simulink model "Test_Model_HR12_2016"  (R2016b)
settings: Solver=FixedStepAuto  StartTime=0.0  StopTime=length(ipoint)  FixedStep=dt  RelTol=1e-3
values from neighbouring files (symbols this model uses):
  Cbx_cyl_fill_efy_intk_mfld_prs_atm_prs_cor_cho = true    [Calib_mdl_RSA.m]
  Cbx_cyl_fill_efy_opt_cho = false    [Calib_mdl_RSA.m]
  Cbx_cyl_fill_igr_opt_cho = false    [Calib_mdl_RSA.m]
  Cbx_ex_vvt_conf = true    [Calib_mdl_RSA.m]
  Cnx_cyl_fill_ex_mfld_prs_cor_cho = 0    [Cal_basic.m]
  Cnx_cyl_nr_conf = 3    [Cal_basic.m]
  Cxx_cyl_fill_efy_drv_max = 20    [Calib_mdl_RSA.m]
  Cxx_cyl_fill_efy_dyn_max = 0.15    [Calib_mdl_RSA.m]
  Cxx_cyl_fill_efy_dyn_min = 0    [Calib_mdl_RSA.m]
  Cxx_cyl_fill_efy_dz = 0.45    [Calib_mdl_RSA.m]
  Cxx_cyl_fill_efy_ovlp_angl = 66    [Calib_mdl_RSA.m]
  Cxx_cyl_fill_efy_vvt_ofs = 0    [Calib_mdl_RSA.m]
  Cxx_cyl_fill_trap_area_h_thd = 0.2    [Cal_basic.m]
  Cxx_cyl_fill_trap_area_l_thd = 0.1    [Cal_basic.m]
  Cxx_cyl_fill_trap_efy_dz_l_thd = 1    [Cal_basic.m]
  Cxx_cyl_fill_trap_efy_dz_neg_slop = -0.5    [Cal_basic.m]
  Cxx_cyl_fill_trap_efy_dz_pos_slop = 0.5    [Cal_basic.m]
  Cxx_cyl_fill_trap_vvt_ovlp_angl = 120    [Calib_mdl_RSA.m]
  Cxx_cyl_vol = 3.9961e-04*3    (= 0.00119883)    [Cal_basic.m]    (also in Calib_mdl_RSA.m = 0.00119900004938)
  Cxx_min_cyl_fill_mdl_ex_mfld_prs_rat_cor = 0    [Cal_basic.m]
  Nnx_eng_run_stt = 2    [Calib_mdl_RSA.m]
  Nxx_atm_kpa = 101.3    [Cal_basic.m]
  Nxx_k_degc = 273.15    [Cal_basic.m]
  Nxx_kilo_bas = 1000    [Cal_basic.m]
  Nxx_wht_pgc_j_kg = 287    [Cal_basic.m]
undefined symbols (not defined in the file or in its folder): Cxx_egr_spc_heat, Cxx_thr_spc_heat, docblock, MapFilling_Aspirated
libraries: AEMS_Standard_Library x78, simulink x2
(part 2 of 5)

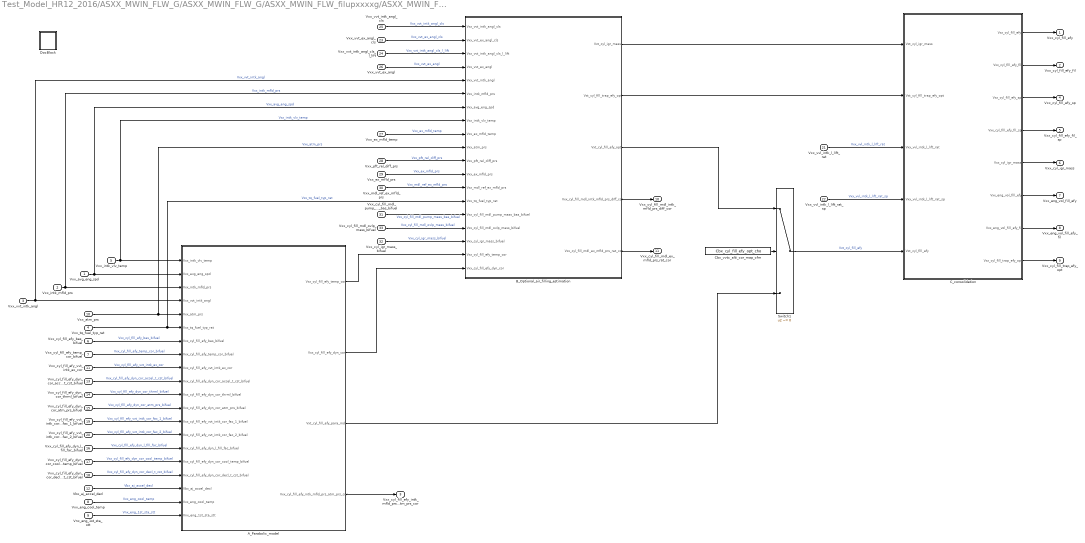
== system Test_Model_HR12_2016/ASXX_MWIN_FLW_G/ASXX_MWIN_FLW_G/ASXX_MWIN_FLW_filupxxxxg/ASXX_MWIN_FLW_filupxxxxg_10ms ==
  Vxx_avg_eng_spd : Inport  Interpolate=off
  Vxx_intk_mfld_prs : Inport  Port=2  Interpolate=off
  Vxx_vvt_intk_angl : Inport  Port=3  Interpolate=off
  Vxx_tq_fuel_typ_rat : Inport  Port=4  Interpolate=off
  Vxx_intk_vlv_temp : Inport  Port=5  Interpolate=off
  Vxx_cyl_fill_efy_bas_bifuel : Inport  Port=6  Interpolate=off
  Vxx_cyl_fill_efy_temp_cor_bifuel : Inport  Port=7  Interpolate=off
  Vxx_eng_cool_temp : Inport  Port=8  Interpolate=off
  Vnx_eng_1st_sta_stt : Inport  Port=9  Interpolate=off
  Vxx_atm_prs : Inport  Port=10  Interpolate=off
  Vxx_cyl_fill_efy_vvt_intk_ex_cor : Inport  Port=11  Interpolate=off
  Vbx_aj_accel_decl : Inport  Port=12  Interpolate=off
  Vxx_cyl_fill_efy_dyn_cor_accel_t_cst_bifuel : Inport  Port=13  Interpolate=off
  Vxx_cyl_fill_efy_dyn_cor_thrml_bifuel : Inport  Port=14  Interpolate=off
  Vxx_cyl_fill_efy_dyn_cor_atm_prs_bifuel : Inport  Port=15  Interpolate=off
  Vxx_cyl_fill_efy_dyn_l_fill_fac_bifuel : Inport  Port=16  Interpolate=off
  Vxx_cyl_fill_efy_dyn_cor_cool_temp_bifuel : Inport  Port=17  Interpolate=off
  Vxx_cyl_fill_efy_dyn_cor_decl_t_cst_bifuel : Inport  Port=18  Interpolate=off
  Vxx_cyl_fill_efy_vvt_intk_cor_fac_1_bifuel : Inport  Port=19  Interpolate=off
  Vxx_cyl_fill_efy_vvt_intk_cor_fac_2_bifuel : Inport  Port=20  Interpolate=off
  Vxx_vvl_intk_l_lift_rat : Inport  Port=21  Interpolate=off
  Vxx_vvl_intk_l_lift_rat_sp : Inport  Port=22  Interpolate=off
  Vxx_vvt_ex_angl_cls : Inport  Port=23  Interpolate=off
  Vxx_vvt_intk_angl_cls_l_lift : Inport  Port=24  Interpolate=off
  Vxx_vvt_intk_angl_cls : Inport  Port=25  Interpolate=off
  Vxx_vvt_ex_angl : Inport  Port=26  Interpolate=off
  Vxx_ex_mfld_temp : Inport  Port=27  Interpolate=off
  Vxx_pft_rel_diff_prs : Inport  Port=28  Interpolate=off
  Vxx_ex_mfld_prs : Inport  Port=29  Interpolate=off
  Vxx_mdl_ref_ex_mfld_prs : Inport  Port=30  Interpolate=off
  Vxx_cyl_fill_mdl_pump_mass_bas_bifuel : Inport  Port=31  Interpolate=off
  Vxx_cyl_igr_mass_bifuel : Inport  Port=32  Interpolate=off
  Vxx_cyl_fill_mdl_ovlp_mass_bifuel : Inport  Port=33  Interpolate=off
  A_Parabolic_model : Subsystem
  B_Optional_air_filling_estimation : Subsystem
  C_consolidation : Subsystem
  Cbx_vvtc_alti_cor_map_cfm : Constant  Value=Cbx_cyl_fill_efy_opt_cho
  DocBlock : Subsystem  mask(DocBlock){ECoderFlag=, DocumentType=Text}
      mask prompts: ECoderFlag "Simulink:blocks:docblockEmbeddedCoderFlagLabel"; DocumentType "Simulink:blocks:docblockDocTypeLabel"
      mask help: Use this block to save long descriptive text with the model. Double-clicking the block will open an editor.
      mask TypeOptions DocumentType: Text | RTF | HTML
      mask Display:
      | plot([.8 0 0 1 1 .8 .8 1],[1 1 0 0 .8 1 .8 .8]);
      | text(.5,.6,'DOC','horizontalalignment','center');
      | text(.95,.05,get_param(gcb,'DocumentType'),'verticalalignment','bottom','horizontalalignment','right');
  Switch1 : Switch  Criteria=u2 ~= 0  RndMeth=Zero  SaturateOnIntegerOverflow=on  InputSameDT=on
      settings: AttributesFormatString=Criteria=%<Criteria>
  Vxx_cyl_fill_efy : Outport  InitialOutput=1
      settings: AttributesFormatString=<initial=%<InitialOutput>>\n<whendisabled=%<OutputWhenDisabled>>
  Vxx_cyl_fill_efy_fil : Outport  Port=2  InitialOutput=1
      settings: AttributesFormatString=<initial=%<InitialOutput>>\n<whendisabled=%<OutputWhenDisabled>>
  Vxx_cyl_fill_efy_intk_mfld_prs_atm_prs_cor : Outport  Port=3  InitialOutput=101.3
      settings: AttributesFormatString=<initial=%<InitialOutput>>\n<whendisabled=%<OutputWhenDisabled>>
  Vxx_cyl_fill_efy_sp : Outport  Port=4  InitialOutput=1
      settings: AttributesFormatString=<initial=%<InitialOutput>>\n<whendisabled=%<OutputWhenDisabled>>
  Vxx_cyl_fill_efy_fil_sp : Outport  Port=5  InitialOutput=1
      settings: AttributesFormatString=<initial=%<InitialOutput>>\n<whendisabled=%<OutputWhenDisabled>>
  Vxx_cyl_igr_mass : Outport  Port=6  InitialOutput=0
      settings: AttributesFormatString=<initial=%<InitialOutput>>\n<whendisabled=%<OutputWhenDisabled>>
  Vxx_eng_vol_fill_efy : Outport  Port=7  InitialOutput=1
      settings: AttributesFormatString=<initial=%<InitialOutput>>\n<whendisabled=%<OutputWhenDisabled>>
  Vxx_eng_vol_fill_efy_fil : Outport  Port=8  InitialOutput=1
      settings: AttributesFormatString=<initial=%<InitialOutput>>\n<whendisabled=%<OutputWhenDisabled>>
  Vxx_cyl_fill_trap_efy_opt : Outport  Port=9  InitialOutput=1
      settings: AttributesFormatString=<initial=%<InitialOutput>>\n<whendisabled=%<OutputWhenDisabled>>
  Vxx_cyl_fill_mdl_intk_mfld_prs_diff_cor : Outport  Port=10  InitialOutput=0
      settings: AttributesFormatString=<initial=%<InitialOutput>>\n<whendisabled=%<OutputWhenDisabled>>
  Vxx_cyl_fill_mdl_ex_mfld_prs_rat_cor : Outport  Port=11  InitialOutput=1
      settings: AttributesFormatString=<initial=%<InitialOutput>>\n<whendisabled=%<OutputWhenDisabled>>
  wires:
  Cbx_vvtc_alti_cor_map_cfm/1 -> Switch1/2
  Vxx_vvt_ex_angl_cls/1 -> B_Optional_air_filling_estimation/2(Vxx_vvt_ex_angl_cls)  "Vxx_vvt_ex_angl_cls"
  Vxx_vvt_intk_angl_cls_l_lift/1 -> B_Optional_air_filling_estimation/3(Vxx_vvt_intk_angl_cls_l_lift)  "Vxx_vvt_intk_angl_cls_l_lift"
  Vxx_vvt_intk_angl_cls/1 -> B_Optional_air_filling_estimation/1(Vxx_vvt_intk_angl_cls)  "Vxx_vvt_intk_angl_cls"
  Vxx_vvt_ex_angl/1 -> B_Optional_air_filling_estimation/4(Vxx_vvt_ex_angl)  "Vxx_vvt_ex_angl"
  Vxx_avg_eng_spd/1 -> A_Parabolic_model/2(Vxx_avg_eng_spd), B_Optional_air_filling_estimation/7(Vxx_avg_eng_spd)  "Vxx_avg_eng_spd"
  Vxx_intk_mfld_prs/1 -> B_Optional_air_filling_estimation/6(Vxx_intk_mfld_prs), A_Parabolic_model/3(Vxx_intk_mfld_prs)  "Vxx_intk_mfld_prs"
  Vxx_vvt_intk_angl/1 -> B_Optional_air_filling_estimation/5(Vxx_vvt_intk_angl), A_Parabolic_model/4(Vxx_vvt_intk_angl)  "Vxx_vvt_intk_angl"
  Vxx_tq_fuel_typ_rat/1 -> B_Optional_air_filling_estimation/14(Vxx_tq_fuel_typ_rat), A_Parabolic_model/6(Vxx_tq_fuel_typ_rat)  "Vxx_tq_fuel_typ_rat"
  Vxx_intk_vlv_temp/1 -> A_Parabolic_model/1(Vxx_intk_vlv_temp), B_Optional_air_filling_estimation/8(Vxx_intk_vlv_temp)  "Vxx_intk_vlv_temp"
  Vxx_cyl_fill_efy_bas_bifuel/1 -> A_Parabolic_model/7(Vxx_cyl_fill_efy_bas_bifuel)  "Vxx_cyl_fill_efy_bas_bifuel"
  Vxx_cyl_fill_efy_temp_cor_bifuel/1 -> A_Parabolic_model/8(Vxx_cyl_fill_efy_temp_cor_bifuel)  "Vxx_cyl_fill_efy_temp_cor_bifuel"
  Vxx_eng_cool_temp/1 -> A_Parabolic_model/19(Vxx_eng_cool_temp)  "Vxx_eng_cool_temp"
  Vnx_eng_1st_sta_stt/1 -> A_Parabolic_model/20(Vnx_eng_1st_sta_stt)  "Vnx_eng_1st_sta_stt"
  Vxx_atm_prs/1 -> A_Parabolic_model/5(Vxx_atm_prs), B_Optional_air_filling_estimation/10(Vxx_atm_prs)  "Vxx_atm_prs"
  Vxx_cyl_fill_efy_vvt_intk_ex_cor/1 -> A_Parabolic_model/9(Vxx_cyl_fill_efy_vvt_intk_ex_cor)  "Vxx_cyl_fill_efy_vvt_intk_ex_cor"
  Vbx_aj_accel_decl/1 -> A_Parabolic_model/18(Vbx_aj_accel_decl)  "Vbx_aj_accel_decl"
  Vxx_cyl_fill_efy_dyn_cor_accel_t_cst_bifuel/1 -> A_Parabolic_model/10(Vxx_cyl_fill_efy_dyn_cor_accel_t_cst_bifuel)  "Vxx_cyl_fill_efy_dyn_cor_accel_t_cst_bifuel"
  Vxx_cyl_fill_efy_dyn_cor_thrml_bifuel/1 -> A_Parabolic_model/11(Vxx_cyl_fill_efy_dyn_cor_thrml_bifuel)  "Vxx_cyl_fill_efy_dyn_cor_thrml_bifuel"
  Vxx_cyl_fill_efy_dyn_cor_atm_prs_bifuel/1 -> A_Parabolic_model/12(Vxx_cyl_fill_efy_dyn_cor_atm_prs_bifuel)  "Vxx_cyl_fill_efy_dyn_cor_atm_prs_bifuel"
  Vxx_cyl_fill_efy_dyn_l_fill_fac_bifuel/1 -> A_Parabolic_model/15(Vxx_cyl_fill_efy_dyn_l_fill_fac_bifuel)  "Vxx_cyl_fill_efy_dyn_l_fill_fac_bifuel"
  Vxx_cyl_fill_efy_dyn_cor_cool_temp_bifuel/1 -> A_Parabolic_model/16(Vxx_cyl_fill_efy_dyn_cor_cool_temp_bifuel)  "Vxx_cyl_fill_efy_dyn_cor_cool_temp_bifuel"
  Vxx_cyl_fill_efy_dyn_cor_decl_t_cst_bifuel/1 -> A_Parabolic_model/17(Vxx_cyl_fill_efy_dyn_cor_decl_t_cst_bifuel)  "Vxx_cyl_fill_efy_dyn_cor_decl_t_cst_bifuel"
  Vxx_cyl_fill_efy_vvt_intk_cor_fac_1_bifuel/1 -> A_Parabolic_model/13(Vxx_cyl_fill_efy_vvt_intk_cor_fac_1_bifuel)  "Vxx_cyl_fill_efy_vvt_intk_cor_fac_1_bifuel"
  Vxx_cyl_fill_efy_vvt_intk_cor_fac_2_bifuel/1 -> A_Parabolic_model/14(Vxx_cyl_fill_efy_vvt_intk_cor_fac_2_bifuel)  "Vxx_cyl_fill_efy_vvt_intk_cor_fac_2_bifuel"
  A_Parabolic_model/4(Vxx_cyl_fill_efy_intk_mfld_prs_atm_prs_cor) -> Vxx_cyl_fill_efy_intk_mfld_prs_atm_prs_cor/1
  A_Parabolic_model/3(Vxt_cyl_fill_efy_para_mdl) -> Switch1/3
  Switch1/1 -> C_consolidation/5(Vxt_cyl_fill_efy)  "Vxt_cyl_fill_efy"
  Vxx_vvl_intk_l_lift_rat/1 -> C_consolidation/3(Vxx_vvl_intk_l_lift_rat)  "Vxx_vvl_intk_l_lift_rat"
  Vxx_vvl_intk_l_lift_rat_sp/1 -> C_consolidation/4(Vxx_vvl_intk_l_lift_rat_sp)  "Vxx_vvl_intk_l_lift_rat_sp"
  B_Optional_air_filling_estimation/1(Vxt_cyl_igr_mass) -> C_consolidation/1(Vxt_cyl_igr_mass)
  B_Optional_air_filling_estimation/2(Vxt_cyl_fill_trap_efy_opt) -> C_consolidation/2(Vxt_cyl_fill_trap_efy_opt)
  C_consolidation/1(Vxx_cyl_fill_efy) -> Vxx_cyl_fill_efy/1
  C_consolidation/2(Vxx_cyl_fill_efy_fil) -> Vxx_cyl_fill_efy_fil/1
  C_consolidation/3(Vxx_cyl_fill_efy_sp) -> Vxx_cyl_fill_efy_sp/1
  C_consolidation/4(Vxx_cyl_fill_efy_fil_sp) -> Vxx_cyl_fill_efy_fil_sp/1
  C_consolidation/5(Vxx_cyl_igr_mass) -> Vxx_cyl_igr_mass/1
  C_consolidation/6(Vxx_eng_vol_fill_efy) -> Vxx_eng_vol_fill_efy/1
  C_consolidation/7(Vxx_eng_vol_fill_efy_fil) -> Vxx_eng_vol_fill_efy_fil/1
  C_consolidation/8(Vxx_cyl_fill_trap_efy_opt) -> Vxx_cyl_fill_trap_efy_opt/1
  Vxx_ex_mfld_temp/1 -> B_Optional_air_filling_estimation/9(Vxx_ex_mfld_temp)  "Vxx_ex_mfld_temp"
  Vxx_pft_rel_diff_prs/1 -> B_Optional_air_filling_estimation/11(Vxx_pft_rel_diff_prs)  "Vxx_pft_rel_diff_prs"
  Vxx_ex_mfld_prs/1 -> B_Optional_air_filling_estimation/12(Vxx_ex_mfld_prs)  "Vxx_ex_mfld_prs"
  Vxx_mdl_ref_ex_mfld_prs/1 -> B_Optional_air_filling_estimation/13(Vxx_mdl_ref_ex_mfld_prs)  "Vxx_mdl_ref_ex_mfld_prs"
  B_Optional_air_filling_estimation/3(Vxt_cyl_fill_efy_opt) -> Switch1/1
  Vxx_cyl_fill_mdl_pump_mass_bas_bifuel/1 -> B_Optional_air_filling_estimation/15(Vxx_cyl_fill_mdl_pump_mass_bas_bifuel)  "Vxx_cyl_fill_mdl_pump_mass_bas_bifuel"
  Vxx_cyl_fill_mdl_ovlp_mass_bifuel/1 -> B_Optional_air_filling_estimation/16(Vxx_cyl_fill_mdl_ovlp_mass_bifuel)  "Vxx_cyl_fill_mdl_ovlp_mass_bifuel"
  Vxx_cyl_igr_mass_bifuel/1 -> B_Optional_air_filling_estimation/17(Vxx_cyl_igr_mass_bifuel)  "Vxx_cyl_igr_mass_bifuel"
  A_Parabolic_model/2(Vxx_cyl_fill_efy_dyn_cor) -> B_Optional_air_filling_estimation/19(Vxx_cyl_fill_efy_dyn_cor)
  A_Parabolic_model/1(Vxx_cyl_fill_efy_temp_cor) -> B_Optional_air_filling_estimation/18(Vxx_cyl_fill_efy_temp_cor)
  B_Optional_air_filling_estimation/5(Vxx_cyl_fill_mdl_ex_mfld_prs_rat_cor) -> Vxx_cyl_fill_mdl_ex_mfld_prs_rat_cor/1
  B_Optional_air_filling_estimation/4(Vxx_cyl_fill_mdl_intk_mfld_prs_diff_cor) -> Vxx_cyl_fill_mdl_intk_mfld_prs_diff_cor/1

== system Test_Model_HR12_2016/ASXX_MWIN_FLW_G/ASXX_MWIN_FLW_G/ASXX_MWIN_FLW_pumpflwxxg/ASXX_MWIN_FLW_pumpflwxxg_10ms ==
  note: g/s
  note: mg/strk
  note: kg/strk
  Vxx_cyl_fill_efy : Inport  Interpolate=off
  Vxx_min_intk_mfld_prs_pump_flow : Inport  Port=2  Interpolate=off
  Vxx_intk_mfld_prs : Inport  Port=3  Interpolate=off
  Vxx_intk_vlv_temp : Inport  Port=4  Interpolate=off
  Vxx_mgstr_gs_convs : Inport  Port=5  Interpolate=off
  Calibration1 : Constant  Value=1000000  OutDataTypeStr=single
  Cxx_cyl_nr3 : Constant  Value=Cnx_cyl_nr_conf
  Cxx_cyl_vol : Constant  Value=Cxx_cyl_vol
  DocBlock : Subsystem  mask(DocBlock){ECoderFlag=, DocumentType=Text}
      mask prompts: ECoderFlag "Simulink:blocks:docblockEmbeddedCoderFlagLabel"; DocumentType "Simulink:blocks:docblockDocTypeLabel"
      mask help: Use this block to save long descriptive text with the model. Double-clicking the block will open an editor.
      mask TypeOptions DocumentType: Text | RTF | HTML
      mask Display:
      | plot([.8 0 0 1 1 .8 .8 1],[1 1 0 0 .8 1 .8 .8]);
      | text(.5,.6,'DOC','horizontalalignment','center');
      | text(.95,.05,get_param(gcb,'DocumentType'),'verticalalignment','bottom','horizontalalignment','right');
  Nxx_k_degc : Constant  Value=Nxx_k_degc
  Nxx_k_degc1 : Constant  Value=Nxx_kilo_bas
  Nxx_wht_pgc1 : Constant  Value=Nxx_wht_pgc_j_kg
  Product{1..2,4..6,11} (6 alike) : Product  Inputs=**  OutDataTypeStr=Inherit: Inherit via back propagation  RndMeth=Zero
  Product14 : Product  Inputs=/*  OutDataTypeStr=Inherit: Inherit via back propagation  RndMeth=Zero
  Product3 : Product  Inputs=*/  OutDataTypeStr=Inherit: Inherit via back propagation  RndMeth=Zero
  Saturation1 : Saturate  UpperLimit=2000  LowerLimit=0  RndMeth=Zero
      settings: AttributesFormatString=<limits=%<UpperLimit>/%<LowerLimit>>
  Saturation2 : Saturate  UpperLimit=12  LowerLimit=3  RndMeth=Zero
      settings: AttributesFormatString=<limits=%<UpperLimit>/%<LowerLimit>>
  Saturation3 : Saturate  UpperLimit=135794.05  LowerLimit=66914.05  RndMeth=Zero
      settings: AttributesFormatString=<limits=%<UpperLimit>/%<LowerLimit>>
  Sum : Sum  Inputs=+-  OutDataTypeStr=Inherit: Inherit via back propagation  RndMeth=Zero  InputSameDT=on
  Sum3 : Sum  OutDataTypeStr=Inherit: Inherit via back propagation  RndMeth=Zero  InputSameDT=on
  Vxx_cyl_pump_flow : Outport  InitialOutput=0
      settings: AttributesFormatString=<initial=%<InitialOutput>>\n<whendisabled=%<OutputWhenDisabled>>
  wires:
  Vxx_intk_vlv_temp/1 -> Sum3/1  "Vxx_intk_vlv_temp"
  Product14/1 -> Product6/1
  Product1/1 -> Saturation3/1
  Product11/1 -> Product14/2
  Cxx_cyl_vol/1 -> Product3/1
  Product5/1 -> Product11/1
  Sum3/1 -> Product1/1
  Nxx_k_degc/1 -> Sum3/2
  Vxx_intk_mfld_prs/1 -> Sum/1  "Vxx_intk_mfld_prs"
  Nxx_wht_pgc1/1 -> Product1/2
  Vxx_cyl_fill_efy/1 -> Product5/2  "Vxx_cyl_fill_efy"
  Vxx_min_intk_mfld_prs_pump_flow/1 -> Sum/2  "Vxx_min_intk_mfld_prs_pump_flow"
  Sum/1 -> Product4/1
  Product2/1 -> Saturation1/1
  Saturation1/1 -> Vxx_cyl_pump_flow/1  "Vxx_cyl_pump_flow"
  Calibration1/1 -> Product6/2
  Product6/1 -> Product2/1
  Vxx_mgstr_gs_convs/1 -> Product2/2  "Vxx_mgstr_gs_convs"
  Cxx_cyl_nr3/1 -> Saturation2/1
  Saturation2/1 -> Product3/2
  Product3/1 -> Product11/2
  Product4/1 -> Product5/1
  Nxx_k_degc1/1 -> Product4/2
  Saturation3/1 -> Product14/1  "Vxx_intk_vlv_temp_pgc"

== system Test_Model_HR12_2016/ASXX_MWIN_FLW_G/ASXX_MWIN_FLW_G/ASXX_MWIN_FLW_pzeroxxxxg/ASXX_MWIN_FLW_pzeroxxxxg_10ms ==
  Vxx_avg_eng_spd : Inport  Interpolate=off
  Vxx_intk_mfld_prs : Inport  Port=2  Interpolate=off
  Vxx_atm_prs : Inport  Port=3  Interpolate=off
  Vxx_pft_rel_diff_prs : Inport  Port=4  Interpolate=off
  AEMS_Carto_1D_v01_02 : AEMS_Standard_Library/LOOKUP_TABLES/AEMS_LUT_1D  Tag=[LIB]  map_x=Cxb_cyl_fill_eng_spd  map_z=Cxp_min_intk_mfld_prs_pump_flow
      settings: AttributesFormatString=%<MaskType>\nBkPX=%<map_x>\nLUT=%<map_z>
  AEMS_Carto_2D_v01_02 : AEMS_Standard_Library/LOOKUP_TABLES/AEMS_LUT_2D  Tag=[LIB]  map_x=Cxb_cyl_fill_intk_mfld_prs_2  map_y=Cxb_cyl_fill_eng_spd_2  carto=Cxm_min_intk_mfld_prs_pump_flow_atm_prs_cor
      settings: AttributesFormatString=%<MaskType>\nBkPX=%<map_x>\nBkPY=%<map_y>\nMAP=%<carto>
  Cbx_vvtc_alti_cor_map_cfm : Constant  Value=Cbx_cyl_fill_efy_opt_cho
  Divide : Product  Inputs=**  OutDataTypeStr=Inherit: Inherit via back propagation
  DocBlock : Subsystem  mask(DocBlock){ECoderFlag=, DocumentType=Text}
      mask prompts: ECoderFlag "Simulink:blocks:docblockEmbeddedCoderFlagLabel"; DocumentType "Simulink:blocks:docblockDocTypeLabel"
      mask help: Use this block to save long descriptive text with the model. Double-clicking the block will open an editor.
      mask TypeOptions DocumentType: Text | RTF | HTML
      mask Display:
      | plot([.8 0 0 1 1 .8 .8 1],[1 1 0 0 .8 1 .8 .8]);
      | text(.5,.6,'DOC','horizontalalignment','center');
      | text(.95,.05,get_param(gcb,'DocumentType'),'verticalalignment','bottom','horizontalalignment','right');
  Nxx_atm_hpa : Constant  Value=Nxx_atm_kpa
  Nxx_atm_hpa1 : Constant  Value=10
  Nxx_atm_hpa2 : Constant  Value=0
  Product : Product  OutDataTypeStr=Inherit: Inherit via back propagation  RndMeth=Zero
  Saturation1 : Saturate  UpperLimit=1000  LowerLimit=-1000  RndMeth=Zero
      settings: AttributesFormatString=<limits=%<UpperLimit>/%<LowerLimit>>
  Saturation2 : Saturate  UpperLimit=2000  LowerLimit=0  RndMeth=Zero
      settings: AttributesFormatString=<limits=%<UpperLimit>/%<LowerLimit>>
  Sum : Sum  Inputs=+-  OutDataTypeStr=Inherit: Inherit via back propagation  RndMeth=Zero  InputSameDT=on
  Sum1 : Sum  Inputs=+-  OutDataTypeStr=Inherit: Inherit via back propagation  RndMeth=Zero  InputSameDT=on
  Sum2 : Sum  Inputs=+-  OutDataTypeStr=Inherit: Inherit via back propagation  RndMeth=Zero  InputSameDT=on
  Switch1 : Switch  Criteria=u2 ~= 0  RndMeth=Zero  SaturateOnIntegerOverflow=on  InputSameDT=on
      settings: AttributesFormatString=Criteria=%<Criteria>
  Vxx_min_map_maf : Outport  InitialOutput=80
      settings: AttributesFormatString=<initial=%<InitialOutput>>\n<whendisabled=%<OutputWhenDisabled>>
  Vxx_min_intk_mfld_prs_pump_flow : Outport  Port=2  InitialOutput=8
      settings: AttributesFormatString=<initial=%<InitialOutput>>\n<whendisabled=%<OutputWhenDisabled>>
  wires:
  Vxx_avg_eng_spd/1 -> AEMS_Carto_1D_v01_02/1, AEMS_Carto_2D_v01_02/2  "Vxx_avg_eng_spd"
  AEMS_Carto_2D_v01_02/1 -> Product/2
  AEMS_Carto_1D_v01_02/1 -> Sum/1  "Vxx_min_intk_mfld_prs_pump_flow_nom"
  Product/1 -> Saturation1/1
  Sum/1 -> Saturation2/1
  Saturation1/1 -> Sum/2  "Vxx_ex_prs_atm_prs_cor"
  Vxx_intk_mfld_prs/1 -> AEMS_Carto_2D_v01_02/1  "Vxx_intk_mfld_prs"
  Nxx_atm_hpa/1 -> Sum1/1
  Vxx_atm_prs/1 -> Sum1/2  "Vxx_atm_prs"
  Vxx_pft_rel_diff_prs/1 -> Sum2/2  "Vxx_pft_rel_diff_prs"
  Sum1/1 -> Sum2/1
  Sum2/1 -> Product/1
  Switch1/1 -> Vxx_min_intk_mfld_prs_pump_flow/1, Divide/1  "Vxx_min_intk_mfld_prs_pump_flow"
  Nxx_atm_hpa1/1 -> Divide/2
  Cbx_vvtc_alti_cor_map_cfm/1 -> Switch1/2
  Nxx_atm_hpa2/1 -> Switch1/1
  Saturation2/1 -> Switch1/3  "Vxx_min_intk_mfld_prs_pump_flow_bas"
  Divide/1 -> Vxx_min_map_maf/1  "Vxx_min_map_maf"

== system Test_Model_HR12_2016/ASXX_MWIN_FLW_G/ASXX_MWIN_FLW_G/ASXX_MWIN_FLW_trapexxxxg/ASXX_MWIN_FLW_trapexxxxg_10ms ==
  Vxx_avg_eng_spd : Inport  Interpolate=off
  Vxx_cyl_fill_efy_intk_mfld_prs_atm_prs_cor : Inport  Port=2  Interpolate=off
  Vxx_vvt_intk_angl : Inport  Port=3  Interpolate=off
  Vxx_vvt_ex_angl : Inport  Port=4  Interpolate=off
  Cbx_vvtc_in_angl_ofs : Constant  Value=Cbx_ex_vvt_conf
  DocBlock : Subsystem  mask(DocBlock){ECoderFlag=, DocumentType=RTF}
      mask prompts: ECoderFlag "Simulink:blocks:docblockEmbeddedCoderFlagLabel"; DocumentType "Simulink:blocks:docblockDocTypeLabel"
      mask help: Use this block to save long descriptive text with the model. Double-clicking the block will open an editor.
      mask TypeOptions DocumentType: Text | RTF | HTML
      mask Display:
      | plot([.8 0 0 1 1 .8 .8 1],[1 1 0 0 .8 1 .8 .8]);
      | text(.5,.6,'DOC','horizontalalignment','center');
      | text(.95,.05,get_param(gcb,'DocumentType'),'verticalalignment','bottom','horizontalalignment','right');
  Trapexxxxg : Subsystem  TreatAsAtomicUnit=on
  Vxx_cyl_fill_trap_efy_vvt_intk_ex_cor : Outport  SourceOfInitialOutputValue=Input signal
  wires:
  Vxx_avg_eng_spd/1 -> Trapexxxxg/1(Vxx_avg_eng_spd)  "Vxx_avg_eng_spd"
  Vxx_cyl_fill_efy_intk_mfld_prs_atm_prs_cor/1 -> Trapexxxxg/2(Vxx_cyl_fill_efy_intk_mfld_prs_atm_prs_cor)  "Vxx_cyl_fill_efy_intk_mfld_prs_atm_prs_cor"
  Vxx_vvt_intk_angl/1 -> Trapexxxxg/3(Vxx_vvt_intk_angl)  "Vxx_vvt_intk_angl"
  Vxx_vvt_ex_angl/1 -> Trapexxxxg/4(Vxx_vvt_ex_angl)  "Vxx_vvt_ex_angl"
  Cbx_vvtc_in_angl_ofs/1 -> Trapexxxxg/Enable
  Trapexxxxg/1(Vxx_cyl_fill_trap_efy_vvt_intk_ex_cor) -> Vxx_cyl_fill_trap_efy_vvt_intk_ex_cor/1

== system Test_Model_HR12_2016/ASXX_MWIN_FLW_G/ASXX_MWIN_FLW_G/ASXX_MWIN_FLW_trapinxxxg/ASXX_MWIN_FLW_trapinxxxg_10ms ==
  Vxx_avg_eng_spd : Inport  Interpolate=off
  Vxx_cyl_fill_efy_intk_mfld_prs_atm_prs_cor : Inport  Port=2  Interpolate=off
  Vxx_cyl_fill_trap_efy_vvt_intk_ex_cor : Inport  Port=3  Interpolate=off
  Vxx_cyl_fill_trap_efy_opt : Inport  Port=4  Interpolate=off
  Cbx_vvtc_in_angl_ofs : Constant  Value=Cbx_ex_vvt_conf
  DocBlock : Subsystem  mask(DocBlock){ECoderFlag=, DocumentType=RTF}
      mask prompts: ECoderFlag "Simulink:blocks:docblockEmbeddedCoderFlagLabel"; DocumentType "Simulink:blocks:docblockDocTypeLabel"
      mask help: Use this block to save long descriptive text with the model. Double-clicking the block will open an editor.
      mask TypeOptions DocumentType: Text | RTF | HTML
      mask Display:
      | plot([.8 0 0 1 1 .8 .8 1],[1 1 0 0 .8 1 .8 .8]);
      | text(.5,.6,'DOC','horizontalalignment','center');
      | text(.95,.05,get_param(gcb,'DocumentType'),'verticalalignment','bottom','horizontalalignment','right');
  Trapinxxxg : Subsystem  TreatAsAtomicUnit=on
  Vxx_cyl_fill_trap_efy : Outport  SourceOfInitialOutputValue=Input signal
  Vxx_eng_trap_fill_efy : Outport  Port=2  SourceOfInitialOutputValue=Input signal
  wires:
  Vxx_avg_eng_spd/1 -> Trapinxxxg/1(Vxx_avg_eng_spd)  "Vxx_avg_eng_spd"
  Vxx_cyl_fill_efy_intk_mfld_prs_atm_prs_cor/1 -> Trapinxxxg/2(Vxx_cyl_fill_efy_intk_mfld_prs_atm_prs_cor)  "Vxx_cyl_fill_efy_intk_mfld_prs_atm_prs_cor"
  Vxx_cyl_fill_trap_efy_vvt_intk_ex_cor/1 -> Trapinxxxg/3(Vxx_cyl_fill_trap_efy_vvt_intk_ex_cor)  "Vxx_cyl_fill_trap_efy_vvt_intk_ex_cor"
  Cbx_vvtc_in_angl_ofs/1 -> Trapinxxxg/Enable
  Trapinxxxg/1(Vxx_cyl_fill_trap_efy) -> Vxx_cyl_fill_trap_efy/1
  Vxx_cyl_fill_trap_efy_opt/1 -> Trapinxxxg/4(Vxx_cyl_fill_trap_efy_opt)  "Vxx_cyl_fill_trap_efy_opt"
  Trapinxxxg/2(Vxx_eng_trap_fill_efy) -> Vxx_eng_trap_fill_efy/1

== system Test_Model_HR12_2016/ASXX_MWIN_FLW_G/ASXX_MWIN_FLW_G/ASXX_MWIN_FLW_filupexxxg/ASXX_MWIN_FLW_filupexxxg_10ms/DocBlock ==
  EmptySubsystem : Subsystem

== system Test_Model_HR12_2016/ASXX_MWIN_FLW_G/ASXX_MWIN_FLW_G/ASXX_MWIN_FLW_filupexxxg/ASXX_MWIN_FLW_filupexxxg_10ms/Filupexxxg ==
  Vxx_avg_eng_spd : Inport  Interpolate=off
  Vxx_cyl_fill_efy_intk_mfld_prs_atm_prs_cor_pudt : Inport  Port=2  Interpolate=off
  Vxx_vvt_intk_angl : Inport  Port=3  Interpolate=off
  Vxx_vvt_ex_angl : Inport  Port=4  Interpolate=off
  Vxx_cyl_fill_efy_vvt_ex_cor_fac_1_bifuel : Inport  Port=5  Interpolate=off
  Vxx_cyl_fill_efy_vvt_ex_cor_fac_2_bifuel : Inport  Port=6  Interpolate=off
  Vxx_tq_fuel_typ_rat : Inport  Port=7  Interpolate=off
  Enable : EnablePort
      settings: AttributesFormatString=StatesWhenEnabling = %<StatesWhenEnabling>
  B1_ex_parabolic_correction : Subsystem
  B2_overlap_correction : Subsystem
  Saturation : Saturate  UpperLimit=1  LowerLimit=-1  RndMeth=Zero
      settings: AttributesFormatString=<limits=%<UpperLimit>/%<LowerLimit>>
  Sum : Sum  OutDataTypeStr=Inherit: Inherit via back propagation  RndMeth=Zero  InputSameDT=on
  Vxx_cyl_fill_efy_vvt_intk_ex_cor : Outport  InitialOutput=0
      settings: AttributesFormatString=<initial=%<InitialOutput>>\n<whendisabled=%<OutputWhenDisabled>>
  wires:
  Vxx_vvt_intk_angl/1 -> B2_overlap_correction/3(Vxx_vvt_intk_angl)
  Vxx_cyl_fill_efy_vvt_ex_cor_fac_1_bifuel/1 -> B1_ex_parabolic_correction/4(Vxx_cyl_fill_efy_vvt_ex_cor_fac_1_bifuel)
  Vxx_cyl_fill_efy_vvt_ex_cor_fac_2_bifuel/1 -> B1_ex_parabolic_correction/5(Vxx_cyl_fill_efy_vvt_ex_cor_fac_2_bifuel)
  Vxx_tq_fuel_typ_rat/1 -> B1_ex_parabolic_correction/6(Vxx_tq_fuel_typ_rat)
  B1_ex_parabolic_correction/1(Vxx_cyl_fill_efy_vvt_ex_cor) -> Sum/1
  Vxx_vvt_ex_angl/1 -> B1_ex_parabolic_correction/3(Vxx_vvt_ex_angl), B2_overlap_correction/4(Vxx_vvt_ex_angl)
  Vxx_cyl_fill_efy_intk_mfld_prs_atm_prs_cor_pudt/1 -> B2_overlap_correction/2(Vxx_cyl_fill_efy_intk_mfld_prs_atm_prs_cor_pudt), B1_ex_parabolic_correction/2(Vxx_cyl_fill_efy_intk_mfld_prs_atm_prs_cor_pudt)
  Sum/1 -> Saturation/1
  Saturation/1 -> Vxx_cyl_fill_efy_vvt_intk_ex_cor/1  "Vxx_cyl_fill_efy_vvt_intk_ex_cor"
  B2_overlap_correction/1(Vxx_cyl_fill_efy_vvt_ovlp_cor) -> Sum/2
  Vxx_avg_eng_spd/1 -> B1_ex_parabolic_correction/1(Vxx_avg_eng_spd), B2_overlap_correction/1(Vxx_avg_eng_spd)

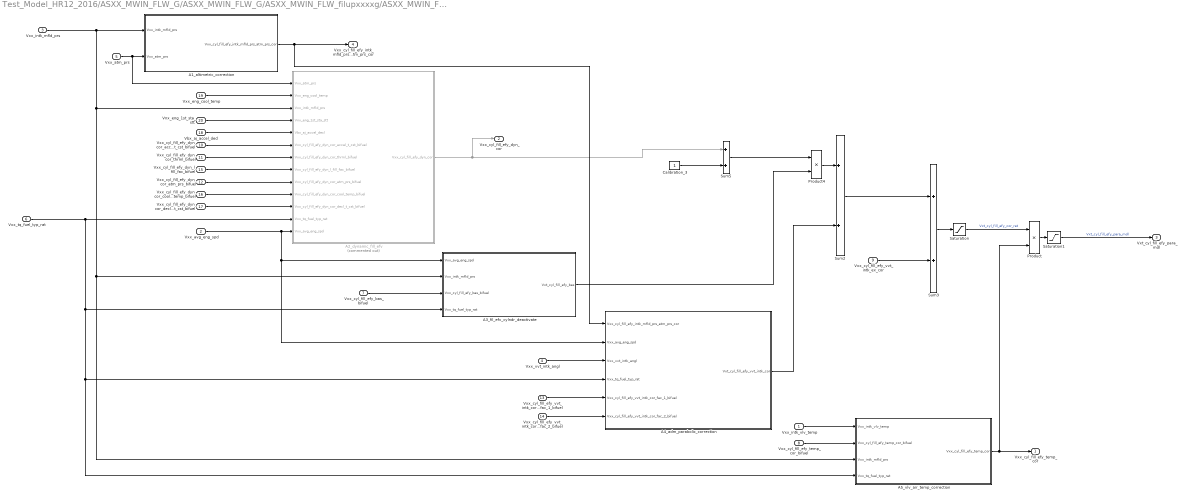
== system Test_Model_HR12_2016/ASXX_MWIN_FLW_G/ASXX_MWIN_FLW_G/ASXX_MWIN_FLW_filupxxxxg/ASXX_MWIN_FLW_filupxxxxg_10ms/A_Parabolic_model ==
  Vxx_intk_vlv_temp : Inport  Interpolate=off
  Vxx_avg_eng_spd : Inport  Port=2  Interpolate=off
  Vxx_intk_mfld_prs : Inport  Port=3  Interpolate=off
  Vxx_vvt_intk_angl : Inport  Port=4  Interpolate=off
  Vxx_atm_prs : Inport  Port=5  Interpolate=off
  Vxx_tq_fuel_typ_rat : Inport  Port=6  Interpolate=off
  Vxx_cyl_fill_efy_bas_bifuel : Inport  Port=7  Interpolate=off
  Vxx_cyl_fill_efy_temp_cor_bifuel : Inport  Port=8  Interpolate=off
  Vxx_cyl_fill_efy_vvt_intk_ex_cor : Inport  Port=9  Interpolate=off
  Vxx_cyl_fill_efy_dyn_cor_accel_t_cst_bifuel : Inport  Port=10  Interpolate=off
  Vxx_cyl_fill_efy_dyn_cor_thrml_bifuel : Inport  Port=11  Interpolate=off
  Vxx_cyl_fill_efy_dyn_cor_atm_prs_bifuel : Inport  Port=12  Interpolate=off
  Vxx_cyl_fill_efy_vvt_intk_cor_fac_1_bifuel : Inport  Port=13  Interpolate=off
  Vxx_cyl_fill_efy_vvt_intk_cor_fac_2_bifuel : Inport  Port=14  Interpolate=off
  Vxx_cyl_fill_efy_dyn_l_fill_fac_bifuel : Inport  Port=15  Interpolate=off
  Vxx_cyl_fill_efy_dyn_cor_cool_temp_bifuel : Inport  Port=16  Interpolate=off
  Vxx_cyl_fill_efy_dyn_cor_decl_t_cst_bifuel : Inport  Port=17  Interpolate=off
  Vbx_aj_accel_decl : Inport  Port=18  Interpolate=off
  Vxx_eng_cool_temp : Inport  Port=19  Interpolate=off
  Vnx_eng_1st_sta_stt : Inport  Port=20  Interpolate=off
  A1_altimetric_correction : Subsystem
  A2_dynamic_fill_efv : Subsystem  Commented=on
  A3_fil_efv_cylndr_deactivate : Subsystem
  A4_adm_parabolic_correction : Subsystem
  A5_vlv_air_temp_correction : Subsystem
  Calibration_3 : Constant
  Product : Product  Inputs=**  OutDataTypeStr=Inherit: Inherit via back propagation  RndMeth=Zero
  Product4 : Product  Inputs=**  OutDataTypeStr=Inherit: Inherit via back propagation  RndMeth=Zero
  Saturation : Saturate  UpperLimit=2  LowerLimit=0  RndMeth=Zero
      settings: AttributesFormatString=<limits=%<UpperLimit>/%<LowerLimit>>
  Saturation1 : Saturate  UpperLimit=2  LowerLimit=0  RndMeth=Zero
      settings: AttributesFormatString=<limits=%<UpperLimit>/%<LowerLimit>>
  Sum2 : Sum  OutDataTypeStr=Inherit: Inherit via back propagation  RndMeth=Zero  InputSameDT=on
  Sum3 : Sum  OutDataTypeStr=Inherit: Inherit via back propagation  RndMeth=Zero  InputSameDT=on
  Sum5 : Sum  OutDataTypeStr=Inherit: Inherit via back propagation  RndMeth=Zero  InputSameDT=on
  Vxx_cyl_fill_efy_temp_cor : Outport
  Vxx_cyl_fill_efy_dyn_cor : Outport  Port=2
  Vxt_cyl_fill_efy_para_mdl : Outport  Port=3
  Vxx_cyl_fill_efy_intk_mfld_prs_atm_prs_cor : Outport  Port=4
  wires:
  Vxx_cyl_fill_efy_dyn_cor_accel_t_cst_bifuel/1 -> A2_dynamic_fill_efv/6(Vxx_cyl_fill_efy_dyn_cor_accel_t_cst_bifuel)
  Vxx_vvt_intk_angl/1 -> A4_adm_parabolic_correction/3(Vxx_vvt_intk_angl)
  Vxx_intk_vlv_temp/1 -> A5_vlv_air_temp_correction/1(Vxx_intk_vlv_temp)
  Vxx_cyl_fill_efy_temp_cor_bifuel/1 -> A5_vlv_air_temp_correction/2(Vxx_cyl_fill_efy_temp_cor_bifuel)
  Vxx_eng_cool_temp/1 -> A2_dynamic_fill_efv/2(Vxx_eng_cool_temp)
  Vnx_eng_1st_sta_stt/1 -> A2_dynamic_fill_efv/4(Vnx_eng_1st_sta_stt)
  Vxx_cyl_fill_efy_bas_bifuel/1 -> A3_fil_efv_cylndr_deactivate/3(Vxx_cyl_fill_efy_bas_bifuel)
  Vxx_cyl_fill_efy_vvt_intk_ex_cor/1 -> Sum3/2
  Vbx_aj_accel_decl/1 -> A2_dynamic_fill_efv/5(Vbx_aj_accel_decl)
  A4_adm_parabolic_correction/1(Vxt_cyl_fill_efy_vvt_intk_cor) -> Sum2/2
  Product4/1 -> Sum2/1
  Vxx_cyl_fill_efy_vvt_intk_cor_fac_2_bifuel/1 -> A4_adm_parabolic_correction/6(Vxx_cyl_fill_efy_vvt_intk_cor_fac_2_bifuel)
  Vxx_intk_mfld_prs/1 -> A5_vlv_air_temp_correction/3(Vxx_intk_mfld_prs), A3_fil_efv_cylndr_deactivate/2(Vxx_intk_mfld_prs), A2_dynamic_fill_efv/3(Vxx_intk_mfld_prs), A1_altimetric_correction/1(Vxx_intk_mfld_prs)
  Saturation/1 -> Product/1  "Vxt_cyl_fill_efy_cor_rat"
  Sum3/1 -> Saturation/1
  Vxx_atm_prs/1 -> A1_altimetric_correction/2(Vxx_atm_prs), A2_dynamic_fill_efv/1(Vxx_atm_prs)
  A3_fil_efv_cylndr_deactivate/1(Vxt_cyl_fill_efy_bas) -> Product4/2
  Vxx_avg_eng_spd/1 -> A3_fil_efv_cylndr_deactivate/1(Vxx_avg_eng_spd), A4_adm_parabolic_correction/2(Vxx_avg_eng_spd), A2_dynamic_fill_efv/13(Vxx_avg_eng_spd)
  Sum2/1 -> Sum3/1
  A2_dynamic_fill_efv/1(Vxx_cyl_fill_efy_dyn_cor) -> Vxx_cyl_fill_efy_dyn_cor/1, Sum5/1
  Vxx_cyl_fill_efy_vvt_intk_cor_fac_1_bifuel/1 -> A4_adm_parabolic_correction/5(Vxx_cyl_fill_efy_vvt_intk_cor_fac_1_bifuel)
  Vxx_cyl_fill_efy_dyn_cor_decl_t_cst_bifuel/1 -> A2_dynamic_fill_efv/11(Vxx_cyl_fill_efy_dyn_cor_decl_t_cst_bifuel)
  Vxx_cyl_fill_efy_dyn_cor_cool_temp_bifuel/1 -> A2_dynamic_fill_efv/10(Vxx_cyl_fill_efy_dyn_cor_cool_temp_bifuel)
  Vxx_cyl_fill_efy_dyn_l_fill_fac_bifuel/1 -> A2_dynamic_fill_efv/8(Vxx_cyl_fill_efy_dyn_l_fill_fac_bifuel)
  Vxx_tq_fuel_typ_rat/1 -> A5_vlv_air_temp_correction/4(Vxx_tq_fuel_typ_rat), A4_adm_parabolic_correction/4(Vxx_tq_fuel_typ_rat), A3_fil_efv_cylndr_deactivate/4(Vxx_tq_fuel_typ_rat), A2_dynamic_fill_efv/12(Vxx_tq_fuel_typ_rat)
  A5_vlv_air_temp_correction/1(Vxx_cyl_fill_efy_temp_cor) -> Vxx_cyl_fill_efy_temp_cor/1, Product/2
  Vxx_cyl_fill_efy_dyn_cor_atm_prs_bifuel/1 -> A2_dynamic_fill_efv/9(Vxx_cyl_fill_efy_dyn_cor_atm_prs_bifuel)
  Vxx_cyl_fill_efy_dyn_cor_thrml_bifuel/1 -> A2_dynamic_fill_efv/7(Vxx_cyl_fill_efy_dyn_cor_thrml_bifuel)
  A1_altimetric_correction/1(Vxx_cyl_fill_efy_intk_mfld_prs_atm_prs_cor) -> Vxx_cyl_fill_efy_intk_mfld_prs_atm_prs_cor/1, A4_adm_parabolic_correction/1(Vxx_cyl_fill_efy_intk_mfld_prs_atm_prs_cor)
  Product/1 -> Saturation1/1
  Saturation1/1 -> Vxt_cyl_fill_efy_para_mdl/1  "Vxt_cyl_fill_efy_para_mdl"
  Calibration_3/1 -> Sum5/2
  Sum5/1 -> Product4/1

== system Test_Model_HR12_2016/ASXX_MWIN_FLW_G/ASXX_MWIN_FLW_G/ASXX_MWIN_FLW_filupxxxxg/ASXX_MWIN_FLW_filupxxxxg_10ms/B_Optional_air_filling_estimation ==
  Vxx_vvt_intk_angl_cls : Inport  Interpolate=off
  Vxx_vvt_ex_angl_cls : Inport  Port=2  Interpolate=off
  Vxx_vvt_intk_angl_cls_l_lift : Inport  Port=3  Interpolate=off
  Vxx_vvt_ex_angl : Inport  Port=4  Interpolate=off
  Vxx_vvt_intk_angl : Inport  Port=5  Interpolate=off
  Vxx_intk_mfld_prs : Inport  Port=6  Interpolate=off
  Vxx_avg_eng_spd : Inport  Port=7  Interpolate=off
  Vxx_intk_vlv_temp : Inport  Port=8  Interpolate=off
  Vxx_ex_mfld_temp : Inport  Port=9  Interpolate=off
  Vxx_atm_prs : Inport  Port=10  Interpolate=off
  Vxx_pft_rel_diff_prs : Inport  Port=11  Interpolate=off
  Vxx_ex_mfld_prs : Inport  Port=12  Interpolate=off
  Vxx_mdl_ref_ex_mfld_prs : Inport  Port=13  Interpolate=off
  Vxx_tq_fuel_typ_rat : Inport  Port=14  Interpolate=off
  Vxx_cyl_fill_mdl_pump_mass_bas_bifuel : Inport  Port=15  Interpolate=off
  Vxx_cyl_fill_mdl_ovlp_mass_bifuel : Inport  Port=16  Interpolate=off
  Vxx_cyl_igr_mass_bifuel : Inport  Port=17  Interpolate=off
  Vxx_cyl_fill_efy_temp_cor : Inport  Port=18  Interpolate=off
  Vxx_cyl_fill_efy_dyn_cor : Inport  Port=19  Interpolate=off
  B1_Pumped_mass_caculation : Subsystem
  B2_Optional_cylinder_filling_efficiency : Subsystem
  B3_Optional_cylinder_trapping_efficiency : Subsystem
  Vxt_cyl_igr_mass : Outport
  Vxt_cyl_fill_trap_efy_opt : Outport  Port=2
  Vxt_cyl_fill_efy_opt : Outport  Port=3
  Vxx_cyl_fill_mdl_intk_mfld_prs_diff_cor : Outport  Port=4
  Vxx_cyl_fill_mdl_ex_mfld_prs_rat_cor : Outport  Port=5
  wires:
  B3_Optional_cylinder_trapping_efficiency/1(Vxt_cyl_fill_trap_efy_opt) -> Vxt_cyl_fill_trap_efy_opt/1
  Vxx_vvt_intk_angl_cls/1 -> B1_Pumped_mass_caculation/3(Vxx_vvt_intk_angl_cls)
  Vxx_vvt_ex_angl_cls/1 -> B1_Pumped_mass_caculation/4(Vxx_vvt_ex_angl_cls)
  Vxx_vvt_intk_angl_cls_l_lift/1 -> B1_Pumped_mass_caculation/5(Vxx_vvt_intk_angl_cls_l_lift)
  Vxx_vvt_intk_angl/1 -> B3_Optional_cylinder_trapping_efficiency/5(Vxx_vvt_intk_angl), B1_Pumped_mass_caculation/7(Vxx_vvt_intk_angl)
  Vxx_intk_mfld_prs/1 -> B1_Pumped_mass_caculation/1(Vxx_intk_mfld_prs), B2_Optional_cylinder_filling_efficiency/1(Vxx_intk_mfld_prs)
  Vxx_avg_eng_spd/1 -> B3_Optional_cylinder_trapping_efficiency/4(Vxx_avg_eng_spd), B1_Pumped_mass_caculation/8(Vxx_avg_eng_spd)
  Vxx_intk_vlv_temp/1 -> B1_Pumped_mass_caculation/2(Vxx_intk_vlv_temp), B2_Optional_cylinder_filling_efficiency/2(Vxx_intk_vlv_temp)
  Vxx_ex_mfld_temp/1 -> B1_Pumped_mass_caculation/9(Vxx_ex_mfld_temp)
  Vxx_atm_prs/1 -> B1_Pumped_mass_caculation/10(Vxx_atm_prs)
  Vxx_pft_rel_diff_prs/1 -> B1_Pumped_mass_caculation/11(Vxx_pft_rel_diff_prs)
  Vxx_ex_mfld_prs/1 -> B1_Pumped_mass_caculation/12(Vxx_ex_mfld_prs)
  Vxx_mdl_ref_ex_mfld_prs/1 -> B1_Pumped_mass_caculation/13(Vxx_mdl_ref_ex_mfld_prs)
  B1_Pumped_mass_caculation/1(Vxt_cyl_fill_mdl_pump_mass) -> B3_Optional_cylinder_trapping_efficiency/1(Vxt_cyl_fill_mdl_pump_mass), B2_Optional_cylinder_filling_efficiency/3(Vxt_cyl_fill_mdl_pump_mass)
  B2_Optional_cylinder_filling_efficiency/1(Vxt_cyl_fill_efy_opt) -> Vxt_cyl_fill_efy_opt/1
  B1_Pumped_mass_caculation/2(Vxt_cyl_fill_mdl_ovlp_mass) -> B3_Optional_cylinder_trapping_efficiency/2(Vxt_cyl_fill_mdl_ovlp_mass)
  Vxx_tq_fuel_typ_rat/1 -> B1_Pumped_mass_caculation/14(Vxx_tq_fuel_typ_rat)
  Vxx_cyl_fill_mdl_pump_mass_bas_bifuel/1 -> B1_Pumped_mass_caculation/15(Vxx_cyl_fill_mdl_pump_mass_bas_bifuel)
  Vxx_cyl_fill_efy_dyn_cor/1 -> B1_Pumped_mass_caculation/19(Vxx_cyl_fill_efy_dyn_cor)
  Vxx_cyl_fill_efy_temp_cor/1 -> B1_Pumped_mass_caculation/16(Vxx_cyl_fill_efy_temp_cor)
  B1_Pumped_mass_caculation/3(Vxt_cyl_igr_mass) -> Vxt_cyl_igr_mass/1
  Vxx_cyl_fill_mdl_ovlp_mass_bifuel/1 -> B1_Pumped_mass_caculation/17(Vxx_cyl_fill_mdl_ovlp_mass_bifuel)
  Vxx_cyl_igr_mass_bifuel/1 -> B1_Pumped_mass_caculation/18(Vxx_cyl_igr_mass_bifuel)
  Vxx_vvt_ex_angl/1 -> B3_Optional_cylinder_trapping_efficiency/6(Vxx_vvt_ex_angl), B1_Pumped_mass_caculation/6(Vxx_vvt_ex_angl)
  B1_Pumped_mass_caculation/4(Vxx_cyl_fill_mdl_intk_mfld_prs_cor) -> B3_Optional_cylinder_trapping_efficiency/3(Vxx_cyl_fill_mdl_intk_mfld_prs_cor)
  B1_Pumped_mass_caculation/6(Vxx_cyl_fill_mdl_ex_mfld_prs_rat_cor) -> Vxx_cyl_fill_mdl_ex_mfld_prs_rat_cor/1
  B1_Pumped_mass_caculation/5(Vxx_cyl_fill_mdl_intk_mfld_prs_diff_cor) -> Vxx_cyl_fill_mdl_intk_mfld_prs_diff_cor/1

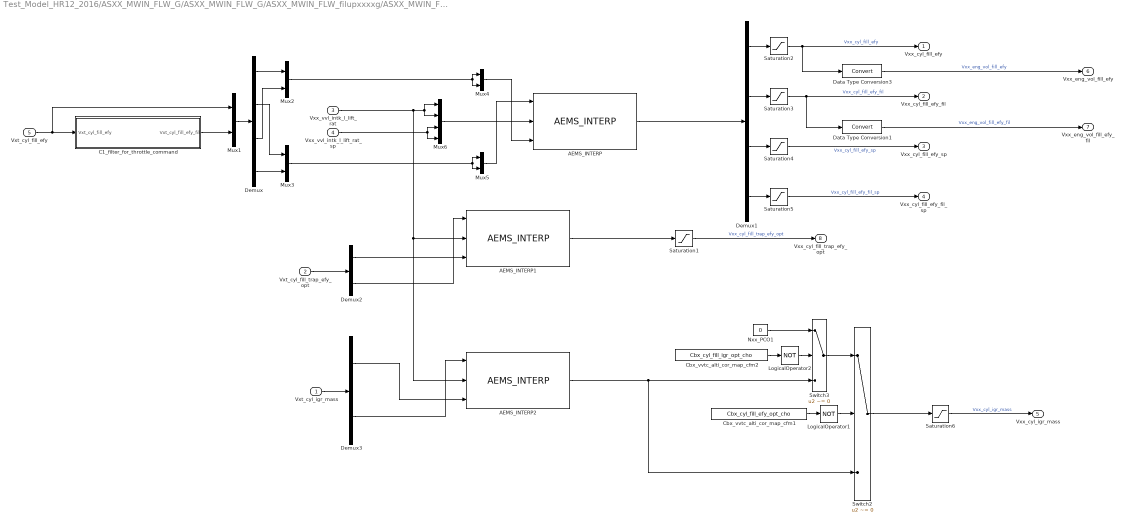
== system Test_Model_HR12_2016/ASXX_MWIN_FLW_G/ASXX_MWIN_FLW_G/ASXX_MWIN_FLW_filupxxxxg/ASXX_MWIN_FLW_filupxxxxg_10ms/C_consolidation ==
  Vxt_cyl_igr_mass : Inport  Interpolate=off
  Vxt_cyl_fill_trap_efy_opt : Inport  Port=2  Interpolate=off
  Vxx_vvl_intk_l_lift_rat : Inport  Port=3  Interpolate=off
  Vxx_vvl_intk_l_lift_rat_sp : Inport  Port=4  Interpolate=off
  Vxt_cyl_fill_efy : Inport  Port=5  Interpolate=off
  AEMS_INTERP : AEMS_Standard_Library/LOOKUP_TABLES/AEMS_INTERP  Tag=[LIB]  Description=This library calculates interpolation for 2 inputs.
      settings: AttributesFormatString=%<MaskType>
  AEMS_INTERP1 : AEMS_Standard_Library/LOOKUP_TABLES/AEMS_INTERP  Tag=[LIB]  Description=This library calculates interpolation for 2 inputs.
      settings: AttributesFormatString=%<MaskType>
  AEMS_INTERP2 : AEMS_Standard_Library/LOOKUP_TABLES/AEMS_INTERP  Tag=[LIB]  Description=This library calculates interpolation for 2 inputs.
      settings: AttributesFormatString=%<MaskType>
  C1_filter_for_throttle_command : Subsystem
  Cbx_vvtc_alti_cor_map_cfm1 : Constant  Value=Cbx_cyl_fill_efy_opt_cho
  Cbx_vvtc_alti_cor_map_cfm2 : Constant  Value=Cbx_cyl_fill_igr_opt_cho
  Data Type Conversion1 : DataTypeConversion
  Data Type Conversion3 : DataTypeConversion
  Demux : Demux
  Demux1 : Demux
  Demux2 : Demux  Outputs=2
  Demux3 : Demux  Outputs=2
  LogicalOperator1 : Logic  Operator=NOT  OutDataTypeStr=boolean
  LogicalOperator2 : Logic  Operator=NOT  OutDataTypeStr=boolean
  Mux{1..5} (5 alike) : Mux  Inputs=2
  Mux6 : Mux
  Nxx_PCO1 : Constant  Value=0
  Saturation{1..5} (5 alike) : Saturate  UpperLimit=2  LowerLimit=0  RndMeth=Zero
      settings: AttributesFormatString=<limits=%<UpperLimit>/%<LowerLimit>>
  Saturation6 : Saturate  UpperLimit=5000  LowerLimit=0  RndMeth=Zero
      settings: AttributesFormatString=<limits=%<UpperLimit>/%<LowerLimit>>
  Switch2 : Switch  Criteria=u2 ~= 0  RndMeth=Zero  SaturateOnIntegerOverflow=on  InputSameDT=on
      settings: AttributesFormatString=Criteria=%<Criteria>
  Switch3 : Switch  Criteria=u2 ~= 0  RndMeth=Zero  SaturateOnIntegerOverflow=on  InputSameDT=on
      settings: AttributesFormatString=Criteria=%<Criteria>
  Vxx_cyl_fill_efy : Outport
  Vxx_cyl_fill_efy_fil : Outport  Port=2
  Vxx_cyl_fill_efy_sp : Outport  Port=3
  Vxx_cyl_fill_efy_fil_sp : Outport  Port=4
  Vxx_cyl_igr_mass : Outport  Port=5
  Vxx_eng_vol_fill_efy : Outport  Port=6
  Vxx_eng_vol_fill_efy_fil : Outport  Port=7
  Vxx_cyl_fill_trap_efy_opt : Outport  Port=8
  wires:
  Mux4/1 -> AEMS_INTERP/3
  Vxt_cyl_fill_efy/1 -> Mux1/1, C1_filter_for_throttle_command/1(Vxt_cyl_fill_efy)
  Demux/1 -> Mux2/1
  C1_filter_for_throttle_command/1(Vxt_cyl_fill_efy_fil) -> Mux1/2
  Demux/4 -> Mux3/2
  Demux/2 -> Mux3/1
  Mux1/1 -> Demux/1
  Demux/3 -> Mux2/2
  Mux2/1 -> Mux4/2, Mux4/1
  Mux3/1 -> Mux5/2, Mux5/1
  Demux2/1 -> AEMS_INTERP1/3
  Demux1/4 -> Saturation5/1
  Vxt_cyl_fill_trap_efy_opt/1 -> Demux2/1
  Vxx_vvl_intk_l_lift_rat_sp/1 -> Mux6/3, Mux6/4
  Switch2/1 -> Saturation6/1
  Demux1/3 -> Saturation4/1
  Saturation3/1 -> Vxx_cyl_fill_efy_fil/1, Data Type Conversion1/1  "Vxx_cyl_fill_efy_fil"
  Mux5/1 -> AEMS_INTERP/1
  Saturation4/1 -> Vxx_cyl_fill_efy_sp/1  "Vxx_cyl_fill_efy_sp"
  Demux2/2 -> AEMS_INTERP1/1
  Saturation2/1 -> Vxx_cyl_fill_efy/1, Data Type Conversion3/1  "Vxx_cyl_fill_efy"
  Saturation5/1 -> Vxx_cyl_fill_efy_fil_sp/1  "Vxx_cyl_fill_efy_fil_sp"
  Demux1/1 -> Saturation2/1
  Mux6/1 -> AEMS_INTERP/2
  Demux1/2 -> Saturation3/1
  Demux3/1 -> AEMS_INTERP2/3
  Demux3/2 -> AEMS_INTERP2/1
  Data Type Conversion3/1 -> Vxx_eng_vol_fill_efy/1  "Vxx_eng_vol_fill_efy"
  Vxx_vvl_intk_l_lift_rat/1 -> AEMS_INTERP2/2, AEMS_INTERP1/2, Mux6/1, Mux6/2
  Vxt_cyl_igr_mass/1 -> Demux3/1
  Data Type Conversion1/1 -> Vxx_eng_vol_fill_efy_fil/1  "Vxx_eng_vol_fill_efy_fil"
  Saturation1/1 -> Vxx_cyl_fill_trap_efy_opt/1  "Vxx_cyl_fill_trap_efy_opt"
  Saturation6/1 -> Vxx_cyl_igr_mass/1  "Vxx_cyl_igr_mass"
  LogicalOperator1/1 -> Switch2/2
  Nxx_PCO1/1 -> Switch3/1
  Cbx_vvtc_alti_cor_map_cfm1/1 -> LogicalOperator1/1
  LogicalOperator2/1 -> Switch3/2
  Switch3/1 -> Switch2/1
  Cbx_vvtc_alti_cor_map_cfm2/1 -> LogicalOperator2/1
  AEMS_INTERP/1 -> Demux1/1
  AEMS_INTERP1/1 -> Saturation1/1
  AEMS_INTERP2/1 -> Switch2/3, Switch3/3

== system Test_Model_HR12_2016/ASXX_MWIN_FLW_G/ASXX_MWIN_FLW_G/ASXX_MWIN_FLW_filupxxxxg/ASXX_MWIN_FLW_filupxxxxg_10ms/DocBlock ==
  EmptySubsystem : Subsystem

== system Test_Model_HR12_2016/ASXX_MWIN_FLW_G/ASXX_MWIN_FLW_G/ASXX_MWIN_FLW_pumpflwxxg/ASXX_MWIN_FLW_pumpflwxxg_10ms/DocBlock ==
  EmptySubsystem : Subsystem

== system Test_Model_HR12_2016/ASXX_MWIN_FLW_G/ASXX_MWIN_FLW_G/ASXX_MWIN_FLW_pzeroxxxxg/ASXX_MWIN_FLW_pzeroxxxxg_10ms/DocBlock ==
  EmptySubsystem : Subsystem

== system Test_Model_HR12_2016/ASXX_MWIN_FLW_G/ASXX_MWIN_FLW_G/ASXX_MWIN_FLW_trapexxxxg/ASXX_MWIN_FLW_trapexxxxg_10ms/DocBlock ==
  EmptySubsystem : Subsystem

== system Test_Model_HR12_2016/ASXX_MWIN_FLW_G/ASXX_MWIN_FLW_G/ASXX_MWIN_FLW_trapexxxxg/ASXX_MWIN_FLW_trapexxxxg_10ms/Trapexxxxg ==
  Vxx_avg_eng_spd : Inport  Interpolate=off
  Vxx_cyl_fill_efy_intk_mfld_prs_atm_prs_cor : Inport  Port=2  Interpolate=off
  Vxx_vvt_intk_angl : Inport  Port=3  Interpolate=off
  Vxx_vvt_ex_angl : Inport  Port=4  Interpolate=off
  Enable : EnablePort
      settings: AttributesFormatString=StatesWhenEnabling = %<StatesWhenEnabling>
  B1_crossing_position_correction : Subsystem
  B2_crossing_angle_correction : Subsystem
  Saturation : Saturate  UpperLimit=1  LowerLimit=-1  RndMeth=Zero
      settings: AttributesFormatString=<limits=%<UpperLimit>/%<LowerLimit>>
  Sum : Sum  Inputs=+-  OutDataTypeStr=Inherit: Inherit via back propagation  RndMeth=Zero  InputSameDT=on
  Vxx_cyl_fill_trap_efy_vvt_intk_ex_cor : Outport  InitialOutput=0
      settings: AttributesFormatString=<initial=%<InitialOutput>>\n<whendisabled=%<OutputWhenDisabled>>
  wires:
  Vxx_vvt_intk_angl/1 -> B1_crossing_position_correction/4(Vxx_vvt_intk_angl), B2_crossing_angle_correction/3(Vxx_vvt_intk_angl)
  Vxx_vvt_ex_angl/1 -> B1_crossing_position_correction/3(Vxx_vvt_ex_angl), B2_crossing_angle_correction/4(Vxx_vvt_ex_angl)
  Sum/1 -> Saturation/1
  Vxx_avg_eng_spd/1 -> B1_crossing_position_correction/1(Vxx_avg_eng_spd), B2_crossing_angle_correction/1(Vxx_avg_eng_spd)
  B1_crossing_position_correction/1(Vxx_cyl_fill_trap_efy_vvt_ovlp_psn_cor) -> Sum/1
  Saturation/1 -> Vxx_cyl_fill_trap_efy_vvt_intk_ex_cor/1  "Vxx_cyl_fill_trap_efy_vvt_intk_ex_cor"
  B2_crossing_angle_correction/1(Vxx_cyl_fill_trap_efy_vvt_ovlp_angl_cor) -> Sum/2
  Vxx_cyl_fill_efy_intk_mfld_prs_atm_prs_cor/1 -> B1_crossing_position_correction/2(Vxx_cyl_fill_efy_intk_mfld_prs_atm_prs_cor), B2_crossing_angle_correction/2(Vxx_cyl_fill_efy_intk_mfld_prs_atm_prs_cor)

== system Test_Model_HR12_2016/ASXX_MWIN_FLW_G/ASXX_MWIN_FLW_G/ASXX_MWIN_FLW_trapinxxxg/ASXX_MWIN_FLW_trapinxxxg_10ms/DocBlock ==
  EmptySubsystem : Subsystem

== system Test_Model_HR12_2016/ASXX_MWIN_FLW_G/ASXX_MWIN_FLW_G/ASXX_MWIN_FLW_trapinxxxg/ASXX_MWIN_FLW_trapinxxxg_10ms/Trapinxxxg ==
  Vxx_avg_eng_spd : Inport  Interpolate=off
  Vxx_cyl_fill_efy_intk_mfld_prs_atm_prs_cor : Inport  Port=2  Interpolate=off
  Vxx_cyl_fill_trap_efy_vvt_intk_ex_cor : Inport  Port=3  Interpolate=off
  Vxx_cyl_fill_trap_efy_opt : Inport  Port=4  Interpolate=off
  Enable : EnablePort
      settings: AttributesFormatString=StatesWhenEnabling = %<StatesWhenEnabling>
  AEMS_Carto_2D_v01_02 : AEMS_Standard_Library/LOOKUP_TABLES/AEMS_LUT_2D  Tag=[LIB]  map_x=Cxb_cyl_fill_eng_spd  map_y=Cxb_cyl_fill_intk_mfld_prs  carto=Cxm_cyl_fill_trap_efy
      settings: AttributesFormatString=%<MaskType>\nBkPX=%<map_x>\nBkPY=%<map_y>\nMAP=%<carto>
  Cbx_vvtc_alti_cor_map_cfm : Constant  Value=Cbx_cyl_fill_efy_opt_cho
  DocBlock : Subsystem  mask(DocBlock){ECoderFlag=, DocumentType=Text}
      mask prompts: ECoderFlag "Simulink:blocks:docblockEmbeddedCoderFlagLabel"; DocumentType "Simulink:blocks:docblockDocTypeLabel"
      mask help: Use this block to save long descriptive text with the model. Double-clicking the block will open an editor.
      mask TypeOptions DocumentType: Text | RTF | HTML
      mask Display:
      | plot([.8 0 0 1 1 .8 .8 1],[1 1 0 0 .8 1 .8 .8]);
      | text(.5,.6,'DOC','horizontalalignment','center');
      | text(.95,.05,get_param(gcb,'DocumentType'),'verticalalignment','bottom','horizontalalignment','right');
  LogicalOperator : Logic  Operator=NOT  OutDataTypeStr=boolean
  Saturation : Saturate  UpperLimit=2  LowerLimit=0  RndMeth=Zero
      settings: AttributesFormatString=<limits=%<UpperLimit>/%<LowerLimit>>
  Saturation1 : Saturate  UpperLimit=2  LowerLimit=0  RndMeth=Zero
      settings: AttributesFormatString=<limits=%<UpperLimit>/%<LowerLimit>>
  Sum3 : Sum  Inputs=2  OutDataTypeStr=Inherit: Inherit via back propagation  RndMeth=Zero  InputSameDT=on
  Switch1 : Switch  Criteria=u2 ~= 0  RndMeth=Zero  SaturateOnIntegerOverflow=on  InputSameDT=on
      settings: AttributesFormatString=Criteria=%<Criteria>
  Vxx_cyl_fill_trap_efy : Outport  InitialOutput=1
      settings: AttributesFormatString=<initial=%<InitialOutput>>\n<whendisabled=%<OutputWhenDisabled>>
  Vxx_eng_trap_fill_efy : Outport  Port=2  InitialOutput=1
      settings: AttributesFormatString=<initial=%<InitialOutput>>\n<whendisabled=%<OutputWhenDisabled>>
  wires:
  Vxx_avg_eng_spd/1 -> AEMS_Carto_2D_v01_02/1
  Vxx_cyl_fill_efy_intk_mfld_prs_atm_prs_cor/1 -> AEMS_Carto_2D_v01_02/2
  Vxx_cyl_fill_trap_efy_vvt_intk_ex_cor/1 -> Sum3/2
  Saturation/1 -> Vxx_cyl_fill_trap_efy/1  "Vxx_cyl_fill_trap_efy"
  Switch1/1 -> Saturation1/1, Saturation/1
  AEMS_Carto_2D_v01_02/1 -> Sum3/1
  Cbx_vvtc_alti_cor_map_cfm/1 -> LogicalOperator/1
  LogicalOperator/1 -> Switch1/2
  Vxx_cyl_fill_trap_efy_opt/1 -> Switch1/3
  Sum3/1 -> Switch1/1
  Saturation1/1 -> Vxx_eng_trap_fill_efy/1  "Vxx_eng_trap_fill_efy"

== system Test_Model_HR12_2016/ASXX_MWIN_FLW_G/ASXX_MWIN_FLW_G/ASXX_MWIN_FLW_filupexxxg/ASXX_MWIN_FLW_filupexxxg_10ms/DocBlock/EmptySubsystem ==
